simulink library "libAtmosphereModel"  (R2020b)
settings: Solver=VariableStepAuto  StartTime=0.0  StopTime=10.0  RelTol=1e-3
settings Model: Creator=caatay  LastModifiedBy=caatay

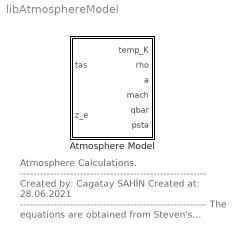
== system libAtmosphereModel ==
  note: Atmosphere Calculations.
      | --------------------------------------------------------
      | Created by: Cagatay SAHİN
      | Created at: 28.06.2021
      | --------------------------------------------------------
      | The equations are obtained from
      | Steven's textbook.
      | The reference book can be found in
      | "references folder".
      | --------------------------------------------------------
      | for question:
      | cagataysahin44@gmail.com
  Atmosphere Model : Subsystem  mask(Environment Model - Atmosphere Model library){lapse_rate=0.703e-5, rho_0=2.377e-3, k=1.4}
      mask prompts: lapse_rate "Lapse Rate"; rho_0 "Sea Level Density"; k "Specific Heat Ratio"
      mask help: International Standar Atmosphere Model in Imerpical Units. The model are obtained with using altitude and true airspeed information.
      mask Help:
      | This block is used for obtain the atmospheric parameters with using state informations.
      | --------------------------------------------------------------------------------------------------------------------------------------------------
      | Input of the function:
      | 	tas: True air speed (ft/s)
      | 	z_e: Altitude (ft)
      | Output of the function:
      | 	t: Temperature (K)
      | 	rho: Density at specific altitıude (slug/ft^3)
      | 	a: Speed of sound at specific altitude (ft/s)
      | 	mach: Mach number ()
      | 	qbar: Dynamic Pressure (lb/ft^2)
      | 	psta: Static Pressure (lb/ft^2)
      | --------------------------------------------------------------------------------------------------------------------------------------------------
      | All equations can be found in Steven's text book. Reference can be found in "literature" subfolder.
      | for question: "cagataysahin44@gmail.com"
      mask Display:
      | port_label('input',1,'V_{tas}','texmode','on');
      | port_label('input',2,'z_{e}','texmode','on');
      | 
      | port_label('output',1,'T_{K}','texmode','on');
      | port_label('output',2,'\rho','texmode','on');
      | port_label('output',3,'a','texmode','on');
      | port_label('output',4,'M','texmode','on');
      | port_label('output',5,'qbar','texmode','on');
      | port_label('output',6,'psta','texmode','on');

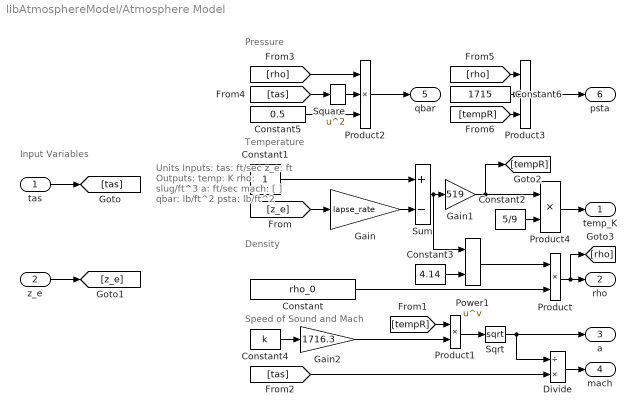
== system libAtmosphereModel/Atmosphere Model ==
  note: Units
      | Inputs:
      | tas: ft/sec
      | z_e: ft
      | Outputs:
      | temp: K
      | rho: slug/ft^3
      | a: ft/sec
      | mach: [ ]
      | qbar: lb/ft^2
      | psta: lb/ft^2
  note: Pressure
  note: Density
  note: Speed of Sound and Mach
  note: Temperature
  note: Input Variables
  "tas " : Inport
  z_e : Inport  Port=2
  Constant : Constant  Value=rho_0
  Constant1 : Constant
  Constant2 : Constant  Value=5/9
  Constant3 : Constant  Value=4.14
  Constant4 : Constant  Value=k
  Constant5 : Constant  Value=0.5
  Constant6 : Constant  Value=1715
  Divide : Product  Inputs=/*
  Gain : Gain  Gain=lapse_rate
  Gain1 : Gain  Gain=519
  Gain2 : Gain  Gain=1716.3
  Power1 : Math  Operator=pow  SignedPower=on  SaturateOnIntegerOverflow=on
  Product : Product
  Product1 : Product
  Product2 : Product  Inputs=3
  Product3 : Product  Inputs=3
  Product4 : Product
  Sqrt : Sqrt  SaturateOnIntegerOverflow=on
  Square : Math  Operator=square  SignedPower=on  SaturateOnIntegerOverflow=on
  Sum : Sum  Inputs=+-
  temp_K : Outport  VectorParamsAs1DForOutWhenUnconnected=off
  rho : Outport  Port=2  VectorParamsAs1DForOutWhenUnconnected=off
  a : Outport  Port=3  VectorParamsAs1DForOutWhenUnconnected=off
  mach : Outport  Port=4  VectorParamsAs1DForOutWhenUnconnected=off
  qbar : Outport  Port=5  VectorParamsAs1DForOutWhenUnconnected=off
  psta : Outport  Port=6  VectorParamsAs1DForOutWhenUnconnected=off
  wires:
  Constant1/1 -> Sum/1
  Product2/1 -> qbar/1
  z_e/1 -> [z_e]
  "tas "/1 -> [tas]
  Sum/1 -> Gain1/1, Power1/1
  Gain/1 -> Sum/2
  Constant/1 -> Product/2
  [z_e] -> Gain/1
  Product4/1 -> temp_K/1
  [tempR] -> Product1/1
  Product/1 -> rho/1, [rho]
  Square/1 -> Product2/2
  Power1/1 -> Product/1
  Gain1/1 -> [tempR], Product4/1
  [rho] -> Product2/1
  Gain2/1 -> Product1/2
  Sqrt/1 -> Divide/1, a/1
  Divide/1 -> mach/1
  [tas] -> Divide/2
  [tempR] -> Product3/3
  Constant2/1 -> Product4/2
  Constant3/1 -> Power1/2
  Product1/1 -> Sqrt/1
  Constant5/1 -> Product2/3
  Constant4/1 -> Gain2/1
  Constant6/1 -> Product3/2
  Product3/1 -> psta/1
  [tas] -> Square/1
  [rho] -> Product3/1
